simulink model "splitting_power_demand"  (R2020a)
settings: Solver=VariableStepAuto  StartTime=0.0  StopTime=1400  RelTol=1e-3
settings Model: Creator=sateeshk  LastModifiedBy=sateeshk

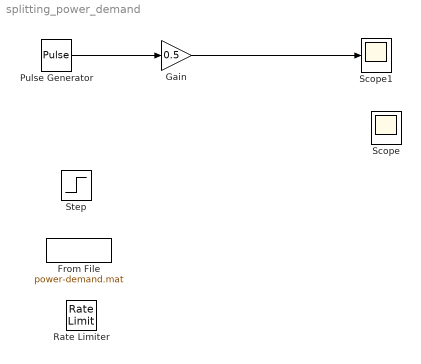
== system splitting_power_demand ==
  From File : FromFile  FileName=power-demand.mat  SampleTime=0
  Gain : Gain  Gain=0.5
  Pulse Generator : DiscretePulseGenerator  PulseType=Time based  Amplitude=400  Period=10  PulseWidth=50
  Rate Limiter : RateLimiter  RisingSlewLimit=300  FallingSlewLimit=-300  SampleTimeMode=inherited
  Scope : Scope  NumInputPorts=2
  Scope1 : Scope
  Step : Step  After=100  SampleTime=0
  wires:
  Gain/1 -> Scope1/1
  Pulse Generator/1 -> Gain/1
